simulink model "ask2"  (Simulink 7.9)
settings: Solver=ode45  StartTime=0.0  StopTime=100  RelTol=1e-3
libraries: commrandsrc2 x1, dsparch4 x1
settings Model: Creator=Abhilash  LastModifiedBy=Yair
settings DebuggingCC: FcnCallInpInsideContextMsg=Use local settings  StrictBusMsg=Warning
settings GRTTargetCC: CombineOutputUpdateFcns=off  GRTInterface=on

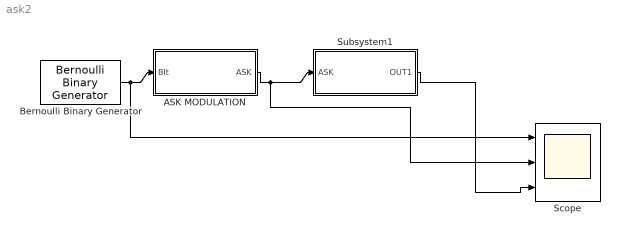
== system ask2 ==
  ASK MODULATION : Subsystem
  Bernoulli Binary Generator : commrandsrc2/Bernoulli Binary Generator  P=0.4  seed=81  Ts=5  frameBased=off  sampPerFrame=1  orient=on  outDataType=double
  Scope : Scope  NumInputPorts=3
      settings: YMin=-5~-5~-5  YMax=5~5~5
  Subsystem1 : Subsystem
  wires:
  ASK MODULATION/1(ASK) -> Subsystem1/1(ASK), Scope/2
  Bernoulli Binary Generator/1 -> ASK MODULATION/1(BIt), Scope/1
  Subsystem1/1(OUT1) -> Scope/3

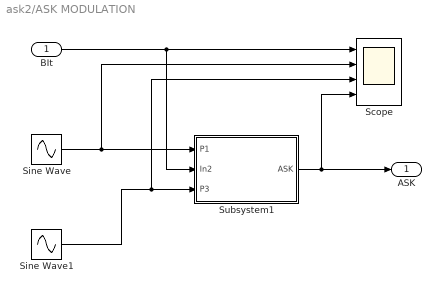
== system ask2/ASK MODULATION ==
  BIt : Inport
  Scope : Scope  NumInputPorts=4
      settings: YMin=-5~-5~-5~-5  YMax=5~5~5~5  SaveName=ScopeData2
  Sine Wave : Sin  SineType=Sample based  Amplitude=2  Samples=50  SampleTime=1/20
  Sine Wave1 : Sin  SineType=Sample based  Amplitude=0.5  Samples=50  SampleTime=1/20
  Subsystem1 : Subsystem
  ASK : Outport
  wires:
  BIt/1 -> Scope/1, Subsystem1/2(In2)
  Sine Wave/1 -> Subsystem1/1(P1), Scope/2
  Sine Wave1/1 -> Subsystem1/3(P3), Scope/3
  Subsystem1/1(ASK) -> ASK/1, Scope/4

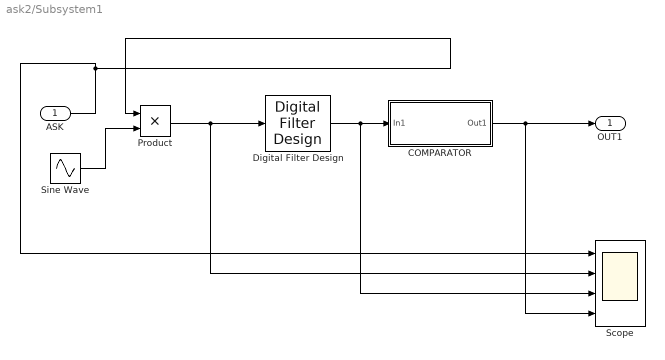
== system ask2/Subsystem1 ==
  ASK : Inport
  COMPARATOR : Subsystem
  Digital Filter Design : dsparch4/Digital Filter Design  mwdsp_browser_bugfix_var=off
  Product : Product  RndMeth=Zero
  Scope : Scope  NumInputPorts=4
      settings: YMin=-5~-5~-5~-5  YMax=5~5~5~5
  Sine Wave : Sin  SineType=Sample based  Samples=50  SampleTime=1/20
  OUT1 : Outport
  wires:
  ASK/1 -> Scope/1, Product/1
  Sine Wave/1 -> Product/2
  COMPARATOR/1(Out1) -> OUT1/1, Scope/4
  Digital Filter Design/1 -> COMPARATOR/1(In1), Scope/3
  Product/1 -> Digital Filter Design/1, Scope/2

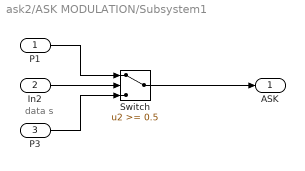
== system ask2/ASK MODULATION/Subsystem1 ==
  note: data s
  P1 : Inport
  In2 : Inport  Port=2
  P3 : Inport  Port=3
  Switch : Switch  Threshold=0.5
  ASK : Outport
  wires:
  P1/1 -> Switch/1
  In2/1 -> Switch/2
  P3/1 -> Switch/3
  Switch/1 -> ASK/1

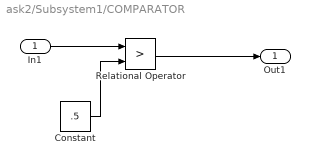
== system ask2/Subsystem1/COMPARATOR ==
  In1 : Inport
  Constant : Constant  Value=.5
  Relational Operator : RelationalOperator  Operator=>  OutDataTypeStr=boolean
  Out1 : Outport
  wires:
  In1/1 -> Relational Operator/1
  Constant/1 -> Relational Operator/2
  Relational Operator/1 -> Out1/1
